simulink model "sl_puma_hw5"  (R2017a)
settings: Solver=ode45  StartTime=0.0  StopTime=time(end-1)  FixedStep=.001  RelTol=1e-3  EnableMultiTasking=on
undefined symbols (not defined in the file or in its folder): time, torque
libraries: roblocks x2
settings Model: ExtModeTrigMode=oneshot  ExtModeArmWhenConnect=off  Creator=pic  LastModifiedBy=jesse
settings DataIOCC: SaveFormat=Array  SignalLoggingSaveFormat=ModelDataLogs  SignalLogging=off  ReturnWorkspaceOutputs=on
settings OptimizationCC: BlockReduction=off  BooleanDataType=off  ExpressionDepthLimit=2147483647  InitFltsAndDblsToZero=on  LifeSpan=inf
settings DebuggingCC: SaveWithParameterizedLinksMsg=none  UnderspecifiedInitializationDetection=Classic  MergeDetectMultiDrivingBlocksExec=none  SignalResolutionControl=TryResolveAllWithWarning  MultiTaskDSMMsg=warning  MultiTaskCondExecSysMsg=none  FcnCallInpInsideContextMsg=warning  StateNameClashWarn=warning  SFUnexpectedBacktrackingDiag=warning  SFNoUnconditionalDefaultTransitionDiag=warning  SFExecutionAtInitializationDiag=none
settings HardwareCC: ProdBitPerPointer=32  ProdBitPerSizeT=32  ProdBitPerPtrDiffT=32  ProdLargestAtomicFloat=None  ProdIntDivRoundTo=Undefined  ProdEndianess=Unspecified  ProdWordSize=32  ProdHWDeviceType=32-bit Generic  TargetUnknown=on
settings ModelReferenceCC: PropagateSignalLabelsOutOfModel=off
settings GRTTargetCC: TargetLangStandard=C89/C90 (ANSI)  ModelReferenceCompliant=off  ParMdlRefBuildCompliant=off  CompOptLevelCompliant=off  GeneratePreprocessorConditionals=Disable all  CombineOutputUpdateFcns=off  MatFileLogging=off  GRTInterface=on
settings ConfigComp: CovMetricSettings=dw  CovHtmlReporting=on  CovSaveCumulativeToWorkspaceVar=on  CovSaveSingleToWorkspaceVar=on  CovExternalEMLEnable=off  CovSFcnEnable=off

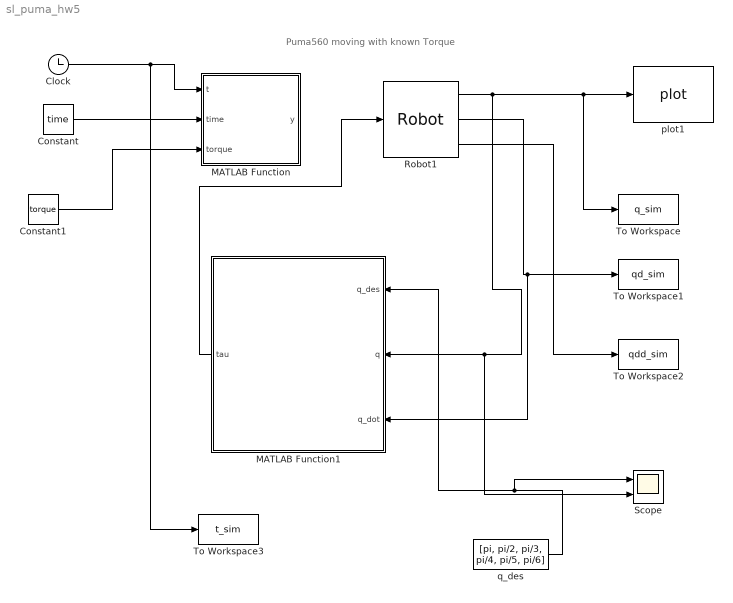
== system sl_puma_hw5 ==
  note: Puma560 moving with known Torque
  Clock : Clock
  Constant : Constant  Value=time
  Constant1 : Constant  Value=torque
  MATLAB Function : MATLAB Function  TreatAsAtomicUnit=on
  MATLAB Function1 : MATLAB Function  TreatAsAtomicUnit=on
  Robot1 : roblocks/Arm/Robot  robot=p560  q0=[0 0 0 0 0 0]
  Scope : Scope  NumInputPorts=2
  To Workspace : ToWorkspace  VariableName=q_sim  SampleTime=-1
  To Workspace1 : ToWorkspace  VariableName=qd_sim  SampleTime=-1
  To Workspace2 : ToWorkspace  VariableName=qdd_sim  SampleTime=-1
  To Workspace3 : ToWorkspace  VariableName=t_sim  SampleTime=-1
  plot1 : roblocks/Arm/plot  robot=p560  fps=5  holdplot=on
  q_des : Constant  Value=[pi, pi/2, pi/3, pi/4, pi/5, pi/6]
  wires:
  Robot1/3 -> To Workspace2/1
  Robot1/2 -> MATLAB Function1/3(q_dot), To Workspace1/1
  Clock/1 -> To Workspace3/1, MATLAB Function/1(t)
  Constant/1 -> MATLAB Function/2(time)
  Constant1/1 -> MATLAB Function/3(torque)
  MATLAB Function1/1(tau) -> Robot1/1
  Robot1/1 -> Scope/2, MATLAB Function1/2(q), plot1/1, To Workspace/1
  q_des/1 -> Scope/1, MATLAB Function1/1(q_des)

== matlab function sl_puma_hw5/MATLAB Function1 ==
  data: q_des input; tau output; q input; q_dot input
function tau = torque_pd_condrol(q_des, q, q_dot)

% q_desired_1 = [pi, pi/2, pi/3, pi/4, pi/5, pi/6];
% q_desired_2 = [pi/6, pi/5, pi/4, pi/3, pi/2, pi];

% kp = 10;
% kd = 2;

kp = [10, 30, 20, 10, 10, 10];
kd = [2, 5, 2, 2, 2, 2];

tau1 = kp(1)*(q_des(1) - q(1)) - kd(1)*(q_dot(1));
tau2 = kp(2)*(q_des(2) - q(2)) - kd(2)*(q_dot(2));
tau3 = kp(3)*(q_des(3) - q(3)) - kd(3)*(q_dot(3));
tau4 = kp(4)*(q_des(4) - q(4)) - kd(4)*(q_dot(4));
tau5 = kp(5)*(q_des(5) - q(5)) - kd(5)*(q_dot(5));
tau6 = kp(6)*(q_des(6) - q(6)) - kd(6)*(q_dot(6));

tau = [tau1, tau2, tau3, tau4, tau5, tau6];
end

== matlab function sl_puma_hw5/MATLAB Function ==
  data: t input; y output; time input; torque input
function y = get_torque(t, time, torque)

y = interp1(time, torque, t);

end
